simulink model "SVPWMProper"  (R2020b)
settings: Solver=ode23t  StartTime=0.0  StopTime=1.5  RelTol=1e-3
libraries: powerlib x49, powerlib_meascontrol x13, pid_lib x4, eePowerMeasurement x4, simulink x2
settings Model: Creator=Matthew  LastModifiedBy=Matthew
settings DataIOCC: ReturnWorkspaceOutputs=off

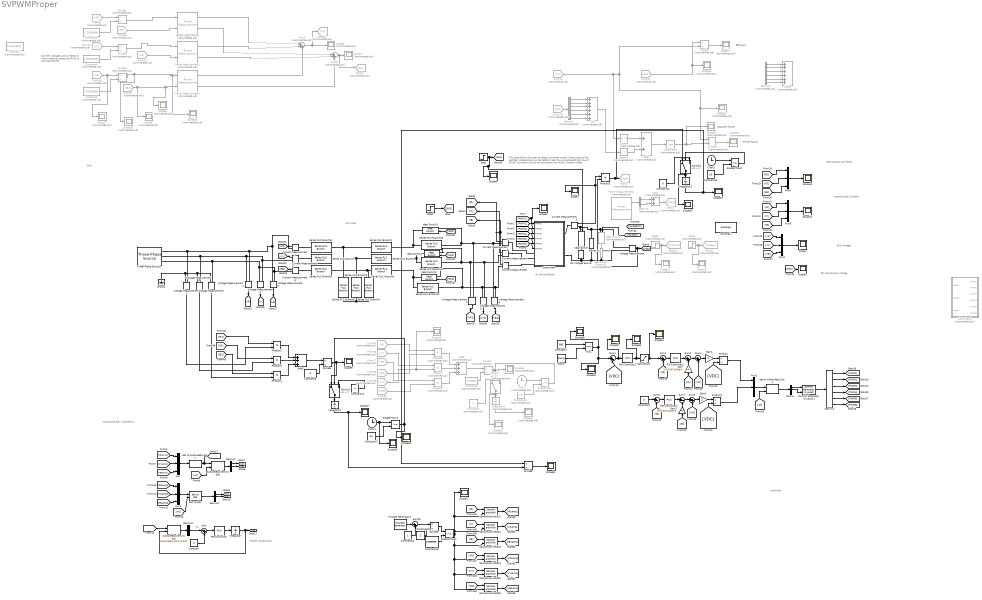
== system SVPWMProper ==
  note: Controller
  note: Phase-Locked
      | Loop
  note: Clarke and Park
      | Transforms
  note: Six-Switch
      | Boost
  note: LCL Filter
  note: Grid
  note: Vq
  note: DC output/input voltage
  note: Grid Voltage
  note: Input/Output Currents
  note: See outputs and inputs
  note: Convert voltages and currents
      | to line-to-neutral values and RMS
      | to calculate power
  note: This step allows the user to select converter mode -
      |  leave step low for rectifier mode and put a step before 0.15s
      | (to simulate settling time of DC/DC converter) to put the converter
      | into DC/DC inverter mode.
  note: Apparent Power
  note: Efficiency
  note: Power Factor
  Add : Sum  Commented=on  Inputs=++++++
  Add1 : Sum  Commented=on
  Add2 : Sum  Commented=on  Inputs=+++
  Add3 : Sum  Inputs=+++
  Add4 : Sum  Commented=on
  Add5 : Sum  Commented=on  Inputs=++++++
  Alpha-Beta-Zero to dq0 : powerlib_meascontrol/Transformations/Alpha-Beta-Zero to dq0  Alignment=90 degrees behind phase A axis
  Alpha-Beta-Zero to dq1 : powerlib_meascontrol/Transformations/Alpha-Beta-Zero to dq0  Alignment=90 degrees behind phase A axis
  Clock : Clock  Commented=on
  Clock1 : Clock
  Clock2 : Clock
  Constant{,2,11,14} (4 alike) : Constant  Value=0
  Constant1 : Constant  Value=800
  Constant10 : Constant  Commented=on  Value=0.5
  Constant12 : Constant  Value=0.5
  Constant13 : Constant  Value=0.5
  Constant24 : Constant
  Constant25 : Constant  Value=2
  Constant26 : Constant  Value=0.999999
  Constant3 : Constant  Commented=on  Value=1.732050808
  Constant4 : Constant  Commented=on  Value=1.732050808
  Constant5 : Constant  Commented=on  Value=1.732050808
  Constant6 : Constant  Value=-1
  Constant7 : Constant  Commented=on  Value=1.414213562
  Constant8 : Constant  Commented=on  Value=-1.73205
  Constant9 : Constant  Commented=on  Value=0
  Current Measurement{,1..6} (7 alike) : powerlib/Measurements/Current Measurement  PhasorSimulation=off  OutputType=Complex  PSBequivalent=0
  DC Voltage Source : powerlib/Electrical Sources/DC Voltage Source  Amplitude=800  Measurements=None
  Demux{,1..3} (4 alike) : Demux  Outputs=3
  Demux4 : Demux  Outputs=6
  Demux5 : Demux  Commented=on  Outputs=6
  Demux6 : Demux  Commented=on  Outputs=2
  Demux7 : Demux  Commented=on  Outputs=6
  Divide{,1..2,4..5,7} (6 alike) : Product  Commented=on  Inputs=*/
  Divide3 : Product  Inputs=*/
  Divide6 : Product  Inputs=*/
  Divide8 : Product  Inputs=*/
  From32 : From  Commented=on  GotoTag=VR
  From33 : From  Commented=on  GotoTag=IR1
  From34 : From  Commented=on  GotoTag=VY
  From35 : From  Commented=on  GotoTag=IY1
  From36 : From  Commented=on  GotoTag=VB
  From37 : From  Commented=on  GotoTag=IB1
  From44 : From  Commented=on  GotoTag=Pin
  From45 : From  Commented=on  GotoTag=Qin
  From47 : From  Commented=on  GotoTag=Pout
  From55 : From  Commented=on  GotoTag=IR
  From56 : From  Commented=on  GotoTag=IY
  From57 : From  Commented=on  GotoTag=IB
  From58 : From  Commented=on  GotoTag=VR1
  From59 : From  Commented=on  GotoTag=VY1
  From60 : From  Commented=on  GotoTag=VB1
  Gain : Gain  Gain=2*pi*50*1000e-6
  Gain1 : Gain  Gain=2
  Gain2 : Gain  Gain=2*pi*50*1000e-6
  Gain3 : Gain  Gain=2
  Goto1 : Goto  Commented=on  GotoTag=Pout
  Goto2 : Goto  Commented=on  GotoTag=Pout
  Goto20 : Goto  Commented=on  GotoTag=SwDefault
  Goto21 : Goto  Commented=on  GotoTag=SwNew
  Goto31 : Goto  Commented=on  GotoTag=Pin
  Goto32 : Goto  Commented=on  GotoTag=Qin
  GreaterThan : RelationalOperator  Commented=on  OutDataTypeStr=boolean  RndMeth=Simplest
  GreaterThan1 : RelationalOperator  OutDataTypeStr=boolean  RndMeth=Simplest
  GreaterThan2 : RelationalOperator  OutDataTypeStr=boolean  RndMeth=Simplest
  GreaterThan3 : RelationalOperator  OutDataTypeStr=boolean  RndMeth=Simplest
  Ground : powerlib/Elements/Ground  LConnTagsString=a
  Ideal Switch : powerlib/Power Electronics/Ideal Switch  Ron=1e-15  Lon=0  IC=0  Rs=inf  Cs=inf  Measurements=off
  Ideal Switch1 : powerlib/Power Electronics/Ideal Switch  Ron=1e-9  Lon=0  IC=0  Rs=inf  Cs=inf  Measurements=off
  Ideal Switch2 : powerlib/Power Electronics/Ideal Switch  Ron=1e-9  Lon=0  IC=0  Rs=inf  Cs=inf  Measurements=off
  Ideal Switch3 : powerlib/Power Electronics/Ideal Switch  Ron=1e-9  Lon=0  IC=0  Rs=inf  Cs=inf  Measurements=off
  Ideal Switch4 : powerlib/Power Electronics/Ideal Switch  Commented=on  Ron=0.001  Lon=0  IC=0  Rs=1e10  Cs=inf  Measurements=off
  Integrator : Integrator
  Integrator1 : Integrator  Commented=on
  Integrator2 : Integrator
  Integrator3 : Integrator
  Min1 : MinMax  Inputs=2
  Mux{,1..5} (6 alike) : Mux  Inputs=3
  PID Controller : pid_lib/PID Controller  Controller=PI  Form=Parallel  TimeDomain=Continuous-time  UseExternalTs=off  SampleTime=-1  IntegratorMethod=Forward Euler  FilterMethod=Forward Euler  ControllerParametersSource=internal  P=10  I=100000  D=0  UseFilter=on  N=100  TunerSelectOption=Transfer Function Based (PID Tuner App)  InitialConditionSource=internal  InitialConditionForIntegrator=0  InitialConditionForFilter=0  DifferentiatorICPrevScaledInput=0  ExternalReset=none  TrackingMode=off  Kt=1  LimitOutput=off  SatLimitsSource=internal  UpperSaturationLimit=inf  LowerSaturationLimit=-inf  LinearizeAsGain=on  AntiWindupMode=none  Kb=1  POutMin=[]  POutMax=[]  IOutMin=[]  IOutMax=[]  DOutMin=[]  DOutMax=[]  NOutMin=[]  NOutMax=[]  SumOutMin=[]  SumOutMax=[]  SaturationOutMin=[]  SaturationOutMax=[]  PParamMin=[]  PParamMax=[]  IParamMin=[]  IParamMax=[]  DParamMin=[]  DParamMax=[]  NParamMin=[]  NParamMax=[]  KbParamMin=[]  KbParamMax=[]  KtParamMin=[]  KtParamMax=[]  KbOutMin=[]  KbOutMax=[]  KtOutMin=[]  KtOutMax=[]  IntegratorOutMin=[]  IntegratorOutMax=[]  FilterOutMin=[]  FilterOutMax=[]  SumI1OutMin=[]  SumI1OutMax=[]  SumI2OutMin=[]  SumI2OutMax=[]  SumI3OutMin=[]  SumI3OutMax=[]  SumI4OutMin=[]  SumI4OutMax=[]  SumDOutMin=[]  SumDOutMax=[]  DifferentiatorOutMin=[]  DifferentiatorOutMax=[]  FilterDiffOutCoefMin=[]  FilterDiffOutCoefMax=[]  ReciprocalOutMin=[]  ReciprocalOutMax=[]  SumDenOutMin=[]  SumDenOutMax=[]  SumNumOutMin=[]  SumNumOutMax=[]  DivideOutMin=[]  DivideOutMax=[]  UdiffTsProdOutMin=[]  UdiffTsProdOutMax=[]  NTsProdOutMin=[]  NTsProdOutMax=[]  UintegralTsProdOutMin=[]  UintegralTsProdOutMax=[]  UngainTsProdOutMin=[]  UngainTsProdOutMax=[]  IntegratorContinuousStateAttributes=''  IntegratorStateMustResolveToSignalObject=off  IntegratorRTWStateStorageClass=Auto  FilterContinuousStateAttributes=''  FilterStateMustResolveToSignalObject=off  FilterRTWStateStorageClass=Auto  ParallelPVariant=InternalParameters  IdealPVariant=Disabled  IVariant=InternalParameters  DVariant=Disabled  IntegratorVariant=Continuous  SatVariant=Disabled  AWVariant=Passthrough  PCopyVariant=Disabled  TRVariant=Disabled  FdbkBlocksVariant=Forward  IdealPFdbkVariant=Disabled  SatFdbkVariant=Disabled  DerivativeFilterVariant=Disabled  NVariant=Disabled  NCopyVariant=Disabled_SignalSpec  FilterICVariant=Disabled  IntegratorICVariant=InternalICs  ExternalResetVariant=Disabled  TRSumVariant=Passthrough  SumFdbkVariant=Disabled  SumVariant=Sum_PI  TsampFilterVariant=InternalTs  TsampNgainVariant=Passthrough  TsampIntegralVariant=Passthrough  ExternalSaturationOutDataTypeStr=Inherit: Same as second input
  PID Controller1 : pid_lib/PID Controller  Controller=PI  Form=Parallel  TimeDomain=Continuous-time  UseExternalTs=off  SampleTime=-1  IntegratorMethod=Forward Euler  FilterMethod=Forward Euler  ControllerParametersSource=internal  P=0.15  I=22  D=0  UseFilter=on  N=100  TunerSelectOption=Transfer Function Based (PID Tuner App)  InitialConditionSource=internal  InitialConditionForIntegrator=0  InitialConditionForFilter=0  DifferentiatorICPrevScaledInput=0  ExternalReset=none  TrackingMode=off  Kt=1  LimitOutput=off  SatLimitsSource=internal  UpperSaturationLimit=inf  LowerSaturationLimit=-inf  LinearizeAsGain=on  AntiWindupMode=none  Kb=1  POutMin=[]  POutMax=[]  IOutMin=[]  IOutMax=[]  DOutMin=[]  DOutMax=[]  NOutMin=[]  NOutMax=[]  SumOutMin=[]  SumOutMax=[]  SaturationOutMin=[]  SaturationOutMax=[]  PParamMin=[]  PParamMax=[]  IParamMin=[]  IParamMax=[]  DParamMin=[]  DParamMax=[]  NParamMin=[]  NParamMax=[]  KbParamMin=[]  KbParamMax=[]  KtParamMin=[]  KtParamMax=[]  KbOutMin=[]  KbOutMax=[]  KtOutMin=[]  KtOutMax=[]  IntegratorOutMin=[]  IntegratorOutMax=[]  FilterOutMin=[]  FilterOutMax=[]  SumI1OutMin=[]  SumI1OutMax=[]  SumI2OutMin=[]  SumI2OutMax=[]  SumI3OutMin=[]  SumI3OutMax=[]  SumI4OutMin=[]  SumI4OutMax=[]  SumDOutMin=[]  SumDOutMax=[]  DifferentiatorOutMin=[]  DifferentiatorOutMax=[]  FilterDiffOutCoefMin=[]  FilterDiffOutCoefMax=[]  ReciprocalOutMin=[]  ReciprocalOutMax=[]  SumDenOutMin=[]  SumDenOutMax=[]  SumNumOutMin=[]  SumNumOutMax=[]  DivideOutMin=[]  DivideOutMax=[]  UdiffTsProdOutMin=[]  UdiffTsProdOutMax=[]  NTsProdOutMin=[]  NTsProdOutMax=[]  UintegralTsProdOutMin=[]  UintegralTsProdOutMax=[]  UngainTsProdOutMin=[]  UngainTsProdOutMax=[]  IntegratorContinuousStateAttributes=''  IntegratorStateMustResolveToSignalObject=off  IntegratorRTWStateStorageClass=Auto  FilterContinuousStateAttributes=''  FilterStateMustResolveToSignalObject=off  FilterRTWStateStorageClass=Auto  ParallelPVariant=InternalParameters  IdealPVariant=Disabled  IVariant=InternalParameters  DVariant=Disabled  IntegratorVariant=Continuous  SatVariant=Disabled  AWVariant=Passthrough  PCopyVariant=Disabled  TRVariant=Disabled  FdbkBlocksVariant=Forward  IdealPFdbkVariant=Disabled  SatFdbkVariant=Disabled  DerivativeFilterVariant=Disabled  NVariant=Disabled  NCopyVariant=Disabled_SignalSpec  FilterICVariant=Disabled  IntegratorICVariant=InternalICs  ExternalResetVariant=Disabled  TRSumVariant=Passthrough  SumFdbkVariant=Disabled  SumVariant=Sum_PI  TsampFilterVariant=InternalTs  TsampNgainVariant=Passthrough  TsampIntegralVariant=Passthrough  ExternalSaturationOutDataTypeStr=Inherit: Same as second input
  PID Controller2 : pid_lib/PID Controller  Controller=PI  Form=Parallel  TimeDomain=Continuous-time  UseExternalTs=off  SampleTime=-1  IntegratorMethod=Forward Euler  FilterMethod=Forward Euler  ControllerParametersSource=internal  P=25  I=500  D=0  UseFilter=on  N=100  TunerSelectOption=Transfer Function Based (PID Tuner App)  InitialConditionSource=internal  InitialConditionForIntegrator=0  InitialConditionForFilter=0  DifferentiatorICPrevScaledInput=0  ExternalReset=none  TrackingMode=off  Kt=1  LimitOutput=off  SatLimitsSource=internal  UpperSaturationLimit=inf  LowerSaturationLimit=-inf  LinearizeAsGain=on  AntiWindupMode=none  Kb=1  POutMin=[]  POutMax=[]  IOutMin=[]  IOutMax=[]  DOutMin=[]  DOutMax=[]  NOutMin=[]  NOutMax=[]  SumOutMin=[]  SumOutMax=[]  SaturationOutMin=[]  SaturationOutMax=[]  PParamMin=[]  PParamMax=[]  IParamMin=[]  IParamMax=[]  DParamMin=[]  DParamMax=[]  NParamMin=[]  NParamMax=[]  KbParamMin=[]  KbParamMax=[]  KtParamMin=[]  KtParamMax=[]  KbOutMin=[]  KbOutMax=[]  KtOutMin=[]  KtOutMax=[]  IntegratorOutMin=[]  IntegratorOutMax=[]  FilterOutMin=[]  FilterOutMax=[]  SumI1OutMin=[]  SumI1OutMax=[]  SumI2OutMin=[]  SumI2OutMax=[]  SumI3OutMin=[]  SumI3OutMax=[]  SumI4OutMin=[]  SumI4OutMax=[]  SumDOutMin=[]  SumDOutMax=[]  DifferentiatorOutMin=[]  DifferentiatorOutMax=[]  FilterDiffOutCoefMin=[]  FilterDiffOutCoefMax=[]  ReciprocalOutMin=[]  ReciprocalOutMax=[]  SumDenOutMin=[]  SumDenOutMax=[]  SumNumOutMin=[]  SumNumOutMax=[]  DivideOutMin=[]  DivideOutMax=[]  UdiffTsProdOutMin=[]  UdiffTsProdOutMax=[]  NTsProdOutMin=[]  NTsProdOutMax=[]  UintegralTsProdOutMin=[]  UintegralTsProdOutMax=[]  UngainTsProdOutMin=[]  UngainTsProdOutMax=[]  IntegratorContinuousStateAttributes=''  IntegratorStateMustResolveToSignalObject=off  IntegratorRTWStateStorageClass=Auto  FilterContinuousStateAttributes=''  FilterStateMustResolveToSignalObject=off  FilterRTWStateStorageClass=Auto  ParallelPVariant=InternalParameters  IdealPVariant=Disabled  IVariant=InternalParameters  DVariant=Disabled  IntegratorVariant=Continuous  SatVariant=Disabled  AWVariant=Passthrough  PCopyVariant=Disabled  TRVariant=Disabled  FdbkBlocksVariant=Forward  IdealPFdbkVariant=Disabled  SatFdbkVariant=Disabled  DerivativeFilterVariant=Disabled  NVariant=Disabled  NCopyVariant=Disabled_SignalSpec  FilterICVariant=Disabled  IntegratorICVariant=InternalICs  ExternalResetVariant=Disabled  TRSumVariant=Passthrough  SumFdbkVariant=Disabled  SumVariant=Sum_PI  TsampFilterVariant=InternalTs  TsampNgainVariant=Passthrough  TsampIntegralVariant=Passthrough  ExternalSaturationOutDataTypeStr=Inherit: Same as second input
  PID Controller4 : pid_lib/PID Controller  Controller=PI  Form=Parallel  TimeDomain=Continuous-time  UseExternalTs=off  SampleTime=-1  IntegratorMethod=Forward Euler  FilterMethod=Forward Euler  ControllerParametersSource=internal  P=25  I=500  D=0  UseFilter=on  N=100  TunerSelectOption=Transfer Function Based (PID Tuner App)  InitialConditionSource=internal  InitialConditionForIntegrator=0  InitialConditionForFilter=0  DifferentiatorICPrevScaledInput=0  ExternalReset=none  TrackingMode=off  Kt=1  LimitOutput=off  SatLimitsSource=internal  UpperSaturationLimit=inf  LowerSaturationLimit=-inf  LinearizeAsGain=on  AntiWindupMode=none  Kb=1  POutMin=[]  POutMax=[]  IOutMin=[]  IOutMax=[]  DOutMin=[]  DOutMax=[]  NOutMin=[]  NOutMax=[]  SumOutMin=[]  SumOutMax=[]  SaturationOutMin=[]  SaturationOutMax=[]  PParamMin=[]  PParamMax=[]  IParamMin=[]  IParamMax=[]  DParamMin=[]  DParamMax=[]  NParamMin=[]  NParamMax=[]  KbParamMin=[]  KbParamMax=[]  KtParamMin=[]  KtParamMax=[]  KbOutMin=[]  KbOutMax=[]  KtOutMin=[]  KtOutMax=[]  IntegratorOutMin=[]  IntegratorOutMax=[]  FilterOutMin=[]  FilterOutMax=[]  SumI1OutMin=[]  SumI1OutMax=[]  SumI2OutMin=[]  SumI2OutMax=[]  SumI3OutMin=[]  SumI3OutMax=[]  SumI4OutMin=[]  SumI4OutMax=[]  SumDOutMin=[]  SumDOutMax=[]  DifferentiatorOutMin=[]  DifferentiatorOutMax=[]  FilterDiffOutCoefMin=[]  FilterDiffOutCoefMax=[]  ReciprocalOutMin=[]  ReciprocalOutMax=[]  SumDenOutMin=[]  SumDenOutMax=[]  SumNumOutMin=[]  SumNumOutMax=[]  DivideOutMin=[]  DivideOutMax=[]  UdiffTsProdOutMin=[]  UdiffTsProdOutMax=[]  NTsProdOutMin=[]  NTsProdOutMax=[]  UintegralTsProdOutMin=[]  UintegralTsProdOutMax=[]  UngainTsProdOutMin=[]  UngainTsProdOutMax=[]  IntegratorContinuousStateAttributes=''  IntegratorStateMustResolveToSignalObject=off  IntegratorRTWStateStorageClass=Auto  FilterContinuousStateAttributes=''  FilterStateMustResolveToSignalObject=off  FilterRTWStateStorageClass=Auto  ParallelPVariant=InternalParameters  IdealPVariant=Disabled  IVariant=InternalParameters  DVariant=Disabled  IntegratorVariant=Continuous  SatVariant=Disabled  AWVariant=Passthrough  PCopyVariant=Disabled  TRVariant=Disabled  FdbkBlocksVariant=Forward  IdealPFdbkVariant=Disabled  SatFdbkVariant=Disabled  DerivativeFilterVariant=Disabled  NVariant=Disabled  NCopyVariant=Disabled_SignalSpec  FilterICVariant=Disabled  IntegratorICVariant=InternalICs  ExternalResetVariant=Disabled  TRSumVariant=Passthrough  SumFdbkVariant=Disabled  SumVariant=Sum_PI  TsampFilterVariant=InternalTs  TsampNgainVariant=Passthrough  TsampIntegralVariant=Passthrough  ExternalSaturationOutDataTypeStr=Inherit: Same as second input
  Power Measurement : eePowerMeasurement/Power Measurement  Commented=on  LabelModeActiveChoice=Continuous  F=50  K=[0 1 2 3 4 5]  Ts=0
      settings: SourceProductBaseCode=PS
  Power Measurement1 : eePowerMeasurement/Power Measurement  Commented=on  LabelModeActiveChoice=Continuous  F=50  K=[0 1 2 3 4 5]  Ts=0
      settings: SourceProductBaseCode=PS
  Power Measurement2 : eePowerMeasurement/Power Measurement  Commented=on  LabelModeActiveChoice=Continuous  F=50  K=[0 1 2 3 4 5]  Ts=0
      settings: SourceProductBaseCode=PS
  Power Measurement3 : eePowerMeasurement/Power Measurement  Commented=on  LabelModeActiveChoice=Continuous  F=50  K=[0 1]  Ts=0
      settings: SourceProductBaseCode=PS
  Product : Product  Inputs=*/
  Product1 : Product  Inputs=*/
  Product{2..5} (4 alike) : Product
  Product6 : Product  Commented=on
  Product7 : Product  Commented=on
  Product8 : Product  Commented=on
  Ramp : simulink/Sources/Ramp  slope=450  start=0  InitialOutput=700
  SVPWM Generator (2-Level)1 : powerlib_meascontrol/Pulse & Signal Generators/SVPWM Generator (2-Level)  InputType=alpha-beta components  SwitchingPattern=Pattern #2  Fc=100e3  ParUref=[0.8 -30 50]  Ts=0
      settings: SourceProductBaseCode=PS
  Sample and Hold{21..26} (6 alike) : powerlib_meascontrol/Additional Components/Sample and Hold  ic=0  Ts=0
      settings: SourceProductBaseCode=PS
  Saturation1 : Saturate  UpperLimit=450  LowerLimit=-240
  Scope{,1..2,5,7,9,11..12,14..15,17,28..29,31..37} (20 alike) : Scope
  Scope{3..4,6,8,10,13,16,18..27,30} (18 alike) : Scope  Commented=on
  Series RLC Branch : powerlib/Elements/Series RLC Branch  LConnTagsString=__new0  RConnTagsString=__new0  BranchType=R  Resistance=6.4  Inductance=1e-3  SetiL0=off  InitialCurrent=0  Capacitance=1e-6  Setx0=off  InitialVoltage=0  Measurements=None
  Series RLC Branch{1..2,5,7..9} (6 alike) : powerlib/Elements/Series RLC Branch  LConnTagsString=__new0  RConnTagsString=__new0  BranchType=RL  Resistance=13.5e-3  Inductance=150e-6  SetiL0=off  InitialCurrent=0  Capacitance=0  Setx0=off  InitialVoltage=0  Measurements=None
  Series RLC Branch10 : powerlib/Elements/Series RLC Branch  LConnTagsString=__new0  RConnTagsString=__new0  BranchType=R  Resistance=1  Inductance=1e-3  SetiL0=off  InitialCurrent=0  Capacitance=1e-6  Setx0=off  InitialVoltage=0  Measurements=None
  Series RLC Branch11 : powerlib/Elements/Series RLC Branch  LConnTagsString=__new0  RConnTagsString=__new0  BranchType=R  Resistance=1  Inductance=1e-3  SetiL0=off  InitialCurrent=0  Capacitance=1e-6  Setx0=off  InitialVoltage=0  Measurements=None
  Series RLC Branch12 : powerlib/Elements/Series RLC Branch  LConnTagsString=__new0  RConnTagsString=__new0  BranchType=R  Resistance=1  Inductance=1e-3  SetiL0=off  InitialCurrent=0  Capacitance=1e-6  Setx0=off  InitialVoltage=0  Measurements=None
  Series RLC Branch13 : powerlib/Elements/Series RLC Branch  Commented=on  LConnTagsString=__new0  RConnTagsString=__new0  BranchType=R  Resistance=5.565  Inductance=1e-3  SetiL0=off  InitialCurrent=0  Capacitance=1e-6  Setx0=off  InitialVoltage=0  Measurements=None
  Series RLC Branch3 : powerlib/Elements/Series RLC Branch  LConnTagsString=__new0  RConnTagsString=__new0  BranchType=RC  Resistance=10e-3  Inductance=1e-3  SetiL0=off  InitialCurrent=0  Capacitance=2e-5  Setx0=off  InitialVoltage=0  Measurements=None
  Series RLC Branch4 : powerlib/Elements/Series RLC Branch  LConnTagsString=__new0  RConnTagsString=__new0  BranchType=RC  Resistance=10e-3  Inductance=1e-3  SetiL0=off  InitialCurrent=0  Capacitance=2e-5  Setx0=off  InitialVoltage=0  Measurements=None
  Series RLC Branch6 : powerlib/Elements/Series RLC Branch  LConnTagsString=__new0  RConnTagsString=__new0  BranchType=RC  Resistance=10e-3  Inductance=1e-3  SetiL0=off  InitialCurrent=0  Capacitance=2e-5  Setx0=off  InitialVoltage=0  Measurements=None
  Square : Math  Commented=on  Operator=square  SaturateOnIntegerOverflow=on
  Square Root : Sqrt  Commented=on  SaturateOnIntegerOverflow=on
  Square1 : Math  Commented=on  Operator=square  SaturateOnIntegerOverflow=on
  Step : Step  Time=10  SampleTime=0
  Step1 : Step  Time=0.02  SampleTime=0
  Step2 : Step  Commented=on  Time=0.6  Before=1  After=0  SampleTime=0
  Step3 : Step  Commented=on  Time=0.6  SampleTime=0
  Subsystem : Subsystem
  Subsystem2 : Subsystem  Commented=on
  Sum : Sum  Inputs=|-+
  Sum{1..2,6..7} (4 alike) : Sum  Inputs=|+-
  Sum{3..4,8,29} (4 alike) : Sum  Inputs=|++
  Sum5 : Sum  Commented=on  Inputs=|+++
  Sum9 : Sum  Commented=on  Inputs=|+++
  Switch : Switch  Commented=on  Criteria=u2 > Threshold
  Switch1 : Switch  Criteria=u2 > Threshold
  Switch2 : Switch  Criteria=u2 > Threshold
  Three-Phase Source1 : powerlib/Electrical Sources/Three-Phase Source  InternalConnection=Yg  VoltagePhases=off  Voltage=400  PhaseAngle=0  Voltage_phases=[25e3 25e3 25e3]/sqrt(3)  PhaseAngles_phases=[0 -120 +120]  Frequency=50  NonIdealSource=on  SpecifyImpedance=off  Resistance=0  Inductance=0  ShortCircuitLevel=100e6  BaseVoltage=400  XRratio=7  BusType=swing  Pref=10e3  Qref=0  Prefabc=[10e3, 10e3, 10e3]  Qrefabc=[0, 0, 0]  Qmin=-inf  Qmax=inf
  Triangle Generator3 : powerlib_meascontrol/Pulse & Signal Generators/Triangle Generator  Freq=100e3  Phase=180  Ts=0
  Voltage Measurement{,1..9} (10 alike) : powerlib/Measurements/Voltage Measurement  PhasorSimulation=off  OutputType=Complex  PSBequivalent=0
  abc to Alpha-Beta-Zero : powerlib_meascontrol/Transformations/abc to Alpha-Beta-Zero
  abc to dq0 : powerlib_meascontrol/Transformations/abc to dq0  Alignment=90 degrees behind phase A axis
  dq0 to Alpha-Beta-Zero : powerlib_meascontrol/Transformations/dq0 to Alpha-Beta-Zero  Alignment=90 degrees behind phase A axis
      settings: SourceProductBaseCode=PS
  powergui : powerlib/powergui  Priority=1  SimulationMode=Discrete  SampleTime=1e-6  frequency=60  Iterations=50  frequencyindice=0  Pbase=100e6  ErrMax=1e-4  UnitsV=kV  UnitsW=MW  buscounter=0  FunctionMessages=off  echomessages=off  EnableUseOfTLC=off  CurrentSourceSwitches=off  DisableSnubberDevices=off  DisableRonSwitches=off  DisableVfSwitches=off  DisplayEquations=off  AutomaticDiscreteSolvers=off  SolverType=Tustin/Backward Euler (TBE)  Interpol=off  ExternalGateDelay=off  methode=off  Ts=100  x0status=blocks  SPID=on  SwTol=0  HookPort=off  NonlinearTolerance=1e-4  nMaxIteration=100  ContinueOnMaxIteration=off  RestoreLinks=warning  ResistiveCurrentMeasurement=off  Frange=[0:2:500]  Ylog=off  Xlog=on  ShowGrid=off  save=off  variable=ZData  structure=Current  ZoomFFT=off  StartTime=1  cycles=10  DisplayStyle=1  fundamental=50  FreqAxis=off  MaxFrequency=200  frequencyindicesteady=1  RmsSteady=1  display=off
  wires:
  Current Measurement2/1 -> [IR]
  Current Measurement1/1 -> [IY]
  Current Measurement/1 -> [IB]
  [PWM1] -> Scope2/1, Subsystem/1(PWM1)
  [PWM2] -> Subsystem/2(PWM2)
  [PWM3] -> Subsystem/3(PWM3)
  [PWM4] -> Subsystem/4(PWM4)
  [PWM5] -> Subsystem/5(PWM5)
  [PWM6] -> Subsystem/6(PWM6)
  [VRsamp] -> Mux/1
  [VBsamp] -> Mux/3
  [VYsamp] -> Mux/2
  Mux/1 -> abc to Alpha-Beta-Zero/1
  abc to Alpha-Beta-Zero/1 -> [alphabeta], Alpha-Beta-Zero to dq0/1
  [wt] -> Alpha-Beta-Zero to dq0/2
  Alpha-Beta-Zero to dq0/1 -> Demux1/1
  Demux1/1 -> [VD]
  Demux1/2 -> [VQ]
  Demux2/2 -> [IQ]
  Demux2/1 -> [ID]
  abc to dq0/1 -> Demux2/1
  Mux1/1 -> abc to dq0/1
  [IYsamp] -> Mux1/2
  [IBsamp] -> Mux1/3
  [IRsamp] -> Mux1/1
  [wt] -> abc to dq0/2
  Alpha-Beta-Zero to dq1/1 -> Demux3/1
  Demux3/2 -> Sum/1
  Constant/1 -> Sum/2
  Sum/1 -> PID Controller/1
  PID Controller/1 -> Integrator/1
  Integrator/1 -> [wt], Alpha-Beta-Zero to dq1/2
  [alphabeta] -> Alpha-Beta-Zero to dq1/1
  [VDC] -> Sum1/2
  Sum1/1 -> Scope37/1, PID Controller1/1
  [ID] -> Sum2/2
  Sum2/1 -> PID Controller2/1
  Gain/1 -> Sum3/2
  PID Controller2/1 -> Sum3/1
  [IQ] -> Gain/1
  Sum3/1 -> Sum4/1
  [VD] -> Sum4/2
  Sum4/1 -> Gain1/1
  Gain1/1 -> Product/1
  [VDC] -> Product/2
  [VDC] -> Product1/2
  Gain3/1 -> Product1/1
  Sum8/1 -> Gain3/1
  [VQ] -> Sum8/2
  Sum7/1 -> Sum8/1
  [ID] -> Gain2/1
  PID Controller4/1 -> Sum7/1
  Gain2/1 -> Sum7/2
  Sum6/1 -> PID Controller4/1
  [IQ] -> Sum6/2
  Constant2/1 -> Sum6/1
  Mux2/1 -> dq0 to Alpha-Beta-Zero/1
  [wt] -> dq0 to Alpha-Beta-Zero/2
  Demux4/1 -> [PWM1]
  Demux4/2 -> [PWM2]
  Demux4/3 -> [PWM3]
  Demux4/4 -> [PWM4]
  Demux4/5 -> [PWM5]
  Demux4/6 -> [PWM6]
  [VR] -> Mux3/1
  [VY] -> Mux3/2
  Mux3/1 -> Scope/1
  [VB] -> Mux3/3
  Mux4/1 -> Scope14/1
  [IY1] -> Mux4/2
  [IB1] -> Mux4/3
  [IR1] -> Mux4/1
  [VDC] -> Scope1/1
  Power Measurement/1 -> Sum5/1
  Power Measurement/2 -> Sum9/1
  Power Measurement1/1 -> Sum5/2
  Power Measurement2/1 -> Sum5/3
  Sum5/1 -> Goto31/1, Scope3/1
  Power Measurement1/2 -> Sum9/2
  Power Measurement2/2 -> Sum9/3
  Sum9/1 -> Goto32/1, Scope4/1
  Sample and Hold25/1 -> [VYsamp]
  [IB] -> Sample and Hold23/1
  Constant26/1 -> GreaterThan3/2
  [VB] -> Sample and Hold26/1
  Sample and Hold23/1 -> [IBsamp]
  Sum29/1 -> Divide3/1
  GreaterThan3/1 -> Scope12/1, Sample and Hold21/2, Sample and Hold22/2, Sample and Hold23/2, Sample and Hold24/2, Sample and Hold25/2, Sample and Hold26/2
  Sample and Hold21/1 -> [IRsamp]
  Divide3/1 -> GreaterThan3/1
  [IY] -> Sample and Hold22/1
  [VY] -> Sample and Hold25/1
  Triangle Generator3/1 -> Sum29/1
  Sample and Hold22/1 -> [IYsamp]
  Constant24/1 -> Sum29/2
  Sample and Hold24/1 -> [VRsamp]
  Sample and Hold26/1 -> [VBsamp]
  Constant25/1 -> Divide3/2
  [VR] -> Sample and Hold24/1
  [IR] -> Sample and Hold21/1
  Ramp/1 -> Min1/2
  Current Measurement4/1 -> [IR1]
  Current Measurement5/1 -> [IY1]
  Current Measurement6/1 -> [IB1]
  Voltage Measurement1/1 -> [VR]
  Voltage Measurement2/1 -> [VY]
  Voltage Measurement3/1 -> [VB]
  Product/1 -> Mux2/1
  Product1/1 -> Mux2/2
  Step/1 -> Ideal Switch/1, Scope9/1, [Sw1]
  [IR] -> Mux5/1
  [IB] -> Mux5/3
  [IY] -> Mux5/2
  Mux5/1 -> Scope11/1
  From45/1 -> Demux7/1
  Demux7/2 -> Add/2
  Demux7/1 -> Add/1
  Demux7/3 -> Add/3
  Demux7/4 -> Add/4
  Demux7/5 -> Add/5
  From44/1 -> Scope22/1, Divide1/1, Divide/2, Square/1
  Demux7/6 -> Add/6
  Add/1 -> Square1/1
  Square/1 -> Add4/1
  Square1/1 -> Add4/2
  Add4/1 -> Square Root/1
  Square Root/1 -> Scope23/1, Divide1/2
  Divide1/1 -> Scope20/1
  Divide/1 -> Scope21/1
  From47/1 -> Scope24/1, Divide/1
  Divide5/1 -> Power Measurement/1
  From33/1 -> Power Measurement/2
  Divide4/1 -> Power Measurement1/1
  From35/1 -> Power Measurement1/2
  From37/1 -> Scope6/1, Power Measurement2/2, Scope8/1
  Divide2/1 -> Scope25/1, Power Measurement2/1, Scope26/1
  From36/1 -> Scope27/1, Divide2/1
  Constant3/1 -> Divide2/2
  From34/1 -> Divide4/1
  Constant4/1 -> Divide4/2
  Constant5/1 -> Divide5/2
  From32/1 -> Divide5/1
  ? -> Subsystem2/1(Varef)
  ? -> Subsystem2/2(Vbref1)
  ? -> Subsystem2/3(Vcref2)
  Demux/1 -> SVPWM Generator (2-Level)1/1
  Demux/2 -> SVPWM Generator (2-Level)1/2
  dq0 to Alpha-Beta-Zero/1 -> Demux/1
  SVPWM Generator (2-Level)1/1 -> Demux4/1
  Demux5/1 -> Add5/1
  Demux5/4 -> Add5/4
  Demux5/2 -> Add5/2
  Demux5/3 -> Add5/3
  Demux5/5 -> Add5/5
  Demux5/6 -> Add5/6
  ? -> Demux5/1
  Constant1/1 -> Min1/1
  PID Controller1/1 -> Scope35/1, Saturation1/1
  Step1/1 -> [SW2]
  [SW2] -> Ideal Switch1/1
  [SW2] -> Ideal Switch2/1
  [SW2] -> Ideal Switch3/1
  Demux6/1 -> Add1/1
  Add1/1 -> Goto2/1
  Demux6/2 -> Add1/2
  Power Measurement3/1 -> Demux6/1
  Voltage Measurement7/1 -> Product2/2
  Voltage Measurement8/1 -> Product3/2
  Voltage Measurement9/1 -> Product4/2
  [IR1] -> Product2/1
  [IY1] -> Product3/1
  [IB1] -> Product4/1
  Product2/1 -> Add3/1
  Product3/1 -> Add3/2
  Product4/1 -> Add3/3
  Add3/1 -> Divide6/1
  Constant6/1 -> Divide6/2
  Divide6/1 -> Switch1/1, Scope5/1
  Product5/1 -> Switch2/1, Goto1/1
  Current Measurement3/1 -> Scope7/1, Product5/1
  Step2/1 -> Goto20/1, Scope10/1
  Step3/1 -> Scope13/1, Goto21/1
  Voltage Measurement/1 -> Product5/2, [VDC]
  [SwNew] -> Ideal Switch4/1
  Min1/1 -> Scope36/1, Scope15/1, Sum1/1
  Voltage Measurement6/1 -> [VB1]
  Voltage Measurement5/1 -> [VY1]
  Voltage Measurement4/1 -> [VR1]
  Divide7/1 -> Switch/1, Scope16/1
  Constant8/1 -> Divide7/2
  Add2/1 -> Divide7/1
  Product8/1 -> Add2/3
  Product7/1 -> Add2/2
  Product6/1 -> Add2/1
  From57/1 -> Product8/1
  From56/1 -> Product7/1
  From55/1 -> Product6/1
  From60/1 -> Product8/2
  From59/1 -> Scope18/1, Product7/2
  From58/1 -> Product6/2
  Clock/1 -> GreaterThan/1
  Constant10/1 -> GreaterThan/2
  Integrator1/1 -> Scope19/1
  Switch/1 -> Scope30/1, Integrator1/1
  GreaterThan/1 -> Switch/2
  Switch1/1 -> Integrator2/1
  Integrator2/1 -> Divide8/2, Scope17/1
  Clock1/1 -> Scope29/1, GreaterThan1/1
  Constant12/1 -> GreaterThan1/2
  GreaterThan1/1 -> Switch1/2, Scope28/1
  Divide8/1 -> Scope31/1
  Constant11/1 -> Switch1/3
  Constant9/1 -> Switch/3
  Switch2/1 -> Scope33/1, Integrator3/1
  Constant14/1 -> Switch2/3
  Integrator3/1 -> Divide8/1, Scope32/1
  Constant13/1 -> GreaterThan2/2
  Clock2/1 -> GreaterThan2/1
  GreaterThan2/1 -> Switch2/2
  Saturation1/1 -> Scope34/1, Sum2/1
  connections:
  Series RLC Branch3/LConn1 -- Series RLC Branch2/RConn1 -- Series RLC Branch7/LConn1
  Series RLC Branch6/LConn1 -- Series RLC Branch1/RConn1 -- Series RLC Branch5/LConn1
  Series RLC Branch6/RConn1 -- Series RLC Branch4/RConn1 -- Series RLC Branch3/RConn1
  Series RLC Branch4/LConn1 -- Series RLC Branch9/RConn1 -- Series RLC Branch8/LConn1
  Current Measurement1/LConn1 -- Subsystem/LConn2
  Subsystem/LConn3 -- Current Measurement/LConn1
  Subsystem/LConn1 -- Current Measurement2/LConn1
  Current Measurement3/RConn1 -- Ideal Switch/LConn1 -- Series RLC Branch/LConn1 -- Ideal Switch4/LConn1 -- Voltage Measurement/LConn1
  Subsystem/RConn2 -- DC Voltage Source/LConn1 -- Series RLC Branch/RConn1 -- Series RLC Branch13/RConn1 -- Voltage Measurement/LConn2
  Current Measurement4/LConn1 -- Series RLC Branch5/RConn1
  Current Measurement5/LConn1 -- Series RLC Branch7/RConn1
  Current Measurement6/LConn1 -- Series RLC Branch8/RConn1
  Voltage Measurement2/LConn1 -- Voltage Measurement8/LConn1 -- Three-Phase Source1/RConn2 -- Voltage Measurement1/LConn2 -- Current Measurement5/RConn1
  Ideal Switch/RConn1 -- DC Voltage Source/RConn1
  Series RLC Branch10/LConn1 -- Series RLC Branch1/LConn1 -- Ideal Switch1/RConn1
  Series RLC Branch9/LConn1 -- Series RLC Branch12/LConn1 -- Ideal Switch3/RConn1
  Series RLC Branch2/LConn1 -- Series RLC Branch11/LConn1 -- Ideal Switch2/RConn1
  Series RLC Branch10/RConn1 -- Ideal Switch1/LConn1 -- Voltage Measurement4/LConn1 -- Voltage Measurement6/LConn2 -- Current Measurement2/RConn1
  Series RLC Branch11/RConn1 -- Ideal Switch2/LConn1 -- Voltage Measurement4/LConn2 -- Voltage Measurement5/LConn1 -- Current Measurement1/RConn1
  Series RLC Branch12/RConn1 -- Ideal Switch3/LConn1 -- Voltage Measurement5/LConn2 -- Voltage Measurement6/LConn1 -- Current Measurement/RConn1
  Current Measurement6/RConn1 -- Voltage Measurement9/LConn1 -- Three-Phase Source1/RConn3 -- Voltage Measurement2/LConn2 -- Voltage Measurement3/LConn1
  Voltage Measurement3/LConn2 -- Voltage Measurement7/LConn1 -- Three-Phase Source1/RConn1 -- Voltage Measurement1/LConn1 -- Current Measurement4/RConn1
  Current Measurement3/LConn1 -- Subsystem/RConn1
  Series RLC Branch13/LConn1 -- Ideal Switch4/RConn1
  Ground/LConn1 -- Voltage Measurement9/LConn2 -- Voltage Measurement8/LConn2 -- Voltage Measurement7/LConn2

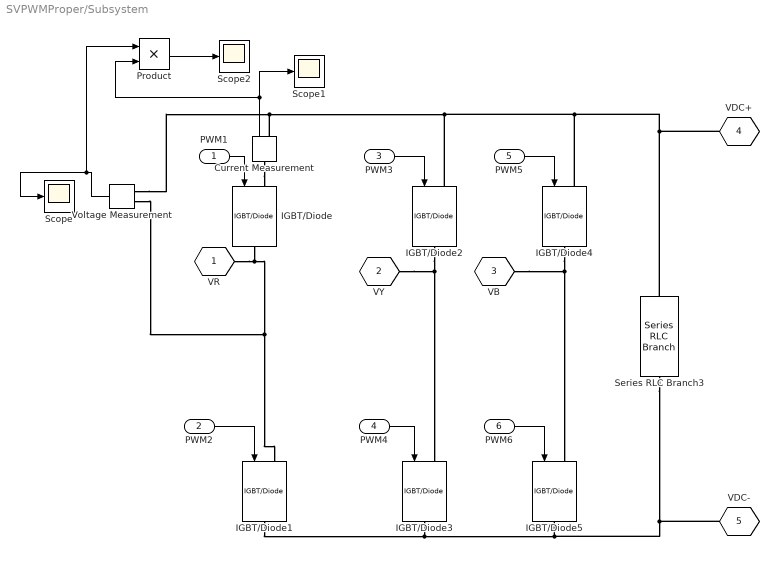
== system SVPWMProper/Subsystem ==
  PWM1 : Inport
  PWM2 : Inport  Port=2
  PWM3 : Inport  Port=3
  PWM4 : Inport  Port=4
  PWM5 : Inport  Port=5
  PWM6 : Inport  Port=6
  Current Measurement : powerlib/Measurements/Current Measurement  PhasorSimulation=off  OutputType=Complex  PSBequivalent=0
  IGBT/Diode{,1..5} (6 alike) : powerlib/Power Electronics/IGBT//Diode  Ron=1e-3  Rs=1e5  Cs=inf  Measurements=off
  Product : Product
  Scope : Scope
  Scope1 : Scope
  Scope2 : Scope
  Series RLC Branch3 : powerlib/Elements/Series RLC Branch  LConnTagsString=__new0  RConnTagsString=__new0  BranchType=RC  Resistance=10e-3  Inductance=1e-3  SetiL0=off  InitialCurrent=0  Capacitance=5.6e-3  Setx0=off  InitialVoltage=0  Measurements=None
  Voltage Measurement : powerlib/Measurements/Voltage Measurement  PhasorSimulation=off  OutputType=Complex  PSBequivalent=0
  VR : PMIOPort  Tag=PMCPort  Side=Left
  VY : PMIOPort  Tag=PMCPort  Port=2  Side=Left
  VB : PMIOPort  Tag=PMCPort  Port=3  Side=Left
  VDC+ : PMIOPort  Tag=PMCPort  Port=4  Side=Right
  VDC- : PMIOPort  Tag=PMCPort  Port=5  Side=Right
  wires:
  PWM2/1 -> IGBT/Diode1/1
  PWM3/1 -> IGBT/Diode2/1
  PWM4/1 -> IGBT/Diode3/1
  PWM6/1 -> IGBT/Diode5/1
  PWM5/1 -> IGBT/Diode4/1
  PWM1/1 -> IGBT/Diode/1
  Voltage Measurement/1 -> Product/1, Scope/1
  Current Measurement/1 -> Product/2, Scope1/1
  Product/1 -> Scope2/1
  connections:
  IGBT/Diode2/LConn1 -- Current Measurement/RConn1 -- Voltage Measurement/LConn1 -- IGBT/Diode4/LConn1 -- Series RLC Branch3/LConn1 -- VDC+/RConn1
  IGBT/Diode4/RConn1 -- VB/RConn1 -- IGBT/Diode5/LConn1
  IGBT/Diode5/RConn1 -- VDC-/RConn1 -- Series RLC Branch3/RConn1 -- IGBT/Diode1/RConn1 -- IGBT/Diode3/RConn1
  IGBT/Diode2/RConn1 -- VY/RConn1 -- IGBT/Diode3/LConn1
  IGBT/Diode/RConn1 -- Voltage Measurement/LConn2 -- IGBT/Diode1/LConn1 -- VR/RConn1
  Current Measurement/LConn1 -- IGBT/Diode/LConn1

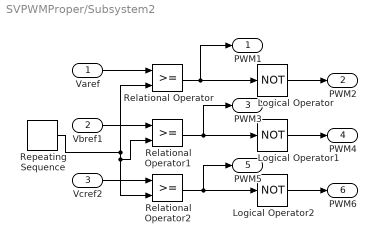
== system SVPWMProper/Subsystem2 ==
  Varef : Inport
  Vbref1 : Inport  Port=2
  Vcref2 : Inport  Port=3
  Logical Operator : Logic  Operator=NOT  AllPortsSameDT=off  OutDataTypeStr=boolean
  Logical Operator1 : Logic  Operator=NOT  AllPortsSameDT=off  OutDataTypeStr=boolean
  Logical Operator2 : Logic  Operator=NOT  AllPortsSameDT=off  OutDataTypeStr=boolean
  Relational Operator : RelationalOperator  OutDataTypeStr=boolean  RndMeth=Simplest
  Relational Operator1 : RelationalOperator  OutDataTypeStr=boolean  RndMeth=Simplest
  Relational Operator2 : RelationalOperator  OutDataTypeStr=boolean  RndMeth=Simplest
  Repeating Sequence : simulink/Sources/Repeating Sequence  rep_seq_t=[0 0.000005 0.00001]  rep_seq_y=[-1 1 -1]
  PWM1 : Outport
  PWM2 : Outport  Port=2
  PWM3 : Outport  Port=3
  PWM4 : Outport  Port=4
  PWM5 : Outport  Port=5
  PWM6 : Outport  Port=6
  wires:
  Varef/1 -> Relational Operator/1
  Logical Operator1/1 -> PWM4/1
  Relational Operator/1 -> Logical Operator/1, PWM1/1
  Relational Operator1/1 -> Logical Operator1/1, PWM3/1
  Repeating Sequence/1 -> Relational Operator/2, Relational Operator1/2, Relational Operator2/2
  Logical Operator/1 -> PWM2/1
  Vbref1/1 -> Relational Operator1/1
  Vcref2/1 -> Relational Operator2/1
  Relational Operator2/1 -> Logical Operator2/1, PWM5/1
  Logical Operator2/1 -> PWM6/1
